simulink model "VOC"  (R2015a)
settings: Solver=ode3  StartTime=0.0  StopTime=3  FixedStep=Ts  RelTol=1e-3
values from neighbouring files (symbols this model uses):
  C = 2350e-6    (= 0.00235)    [VOC_param.m]    (also in VOC_param_paper.m = 0.0022; controller_parameters.m = 0.0022; power_control_param.m)
  Carrier_amp = 10    [VOC_param_paper.m]    (also in controller_parameters.m = 1)
  Ka = fluxeff    (= 0.15)    [VOC_param.m]    (also in VOC_param_paper.m; power_control_param.m)
  Kii = alphaI*R_hat    (= 628.318530718)    [VOC_param_paper.m]    (also in controller_parameters.m; current_controller_param.m = 1260)
  Kiv = 0.01    [VOC_param_paper.m]    (also in controller_parameters.m)
  Kpi = alphaI*L_hat    (= 37.6991118431)    [VOC_param_paper.m]    (also in controller_parameters.m; current_controller_param.m = 62.8)
  Kpv = alphaV*C_hat/(3*Vpcc_hat)    (= 0.0196071030862)    [VOC_param_paper.m]    (also in controller_parameters.m = alphaV*C_hat/(3*Vpcc_hat))
  L = 8e-3    (= 0.008)    [VOC_param.m]    (also in VOC_param_paper.m = 0.003; controller_parameters.m = 0.003; current_controller_param.m = 0.005; power_control_param.m)
  p = 4    [VOC_param.m]    (also in VOC_param_paper.m; power_control_param.m)
  R = 0.1    [VOC_param.m]    (also in VOC_param_paper.m = 0.05; controller_parameters.m = 0.05; current_controller_param.m; power_control_param.m)
  RL = 120    [VOC_param.m]    (also in VOC_param_paper.m = 150; power_control_param.m)
  rpm2radps = pi/30    (= 0.10471975512)    [VOC_param.m]    (also in VOC_param_paper.m; power_control_param.m)
  Ts = 1/fs    (= 1e-05)    [VOC_param.m]    (also in VOC_param_paper.m = 5e-05; controller_parameters.m = 5e-05; power_control_param.m)
  Udcref = 120    [VOC_param.m]    (also in VOC_param_paper.m; power_control_param.m = 100)
libraries: simulink x7, powerlib_meascontrol x6
settings Model: Creator=rblan  LastModifiedBy=rblan

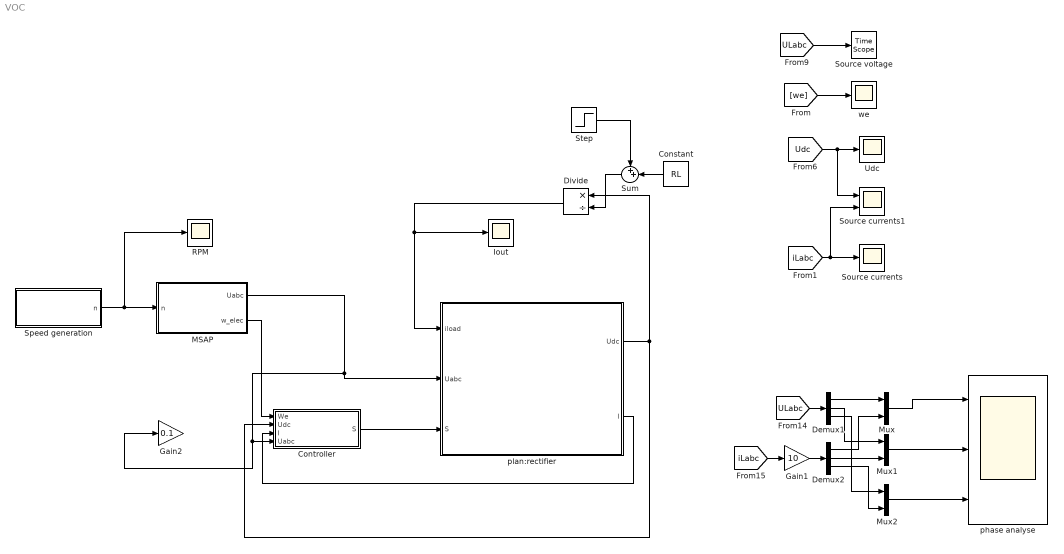
== system VOC ==
  Constant : Constant  Value=RL
  Controller : Subsystem
  Demux1 : Demux  Outputs=3
  Demux2 : Demux  Outputs=3
  Divide : Product  Inputs=*/
  Gain1 : Gain  Gain=10
  Gain2 : Gain  Gain=0.1
  Iout : Scope
      settings: YMin=0.2275  YMax=0.2575
  MSAP : Subsystem
  Mux : Mux  Inputs=2
  Mux1 : Mux  Inputs=2
  Mux2 : Mux  Inputs=2
  RPM : Scope
      settings: YMin=0.2275  YMax=0.2575  SaveName=ScopeData26
  Source currents : Scope
      settings: TimeRange=2  YMin=-11  YMax=11  SaveName=Iabc
  Source currents1 : Scope  NumInputPorts=2
      settings: TimeRange=2  YMin=-11~-5  YMax=11~5  SaveName=Iabc2
  "Source voltage " : TimeScope
  Speed generation : Subsystem
  Step : Step  Time=0.5  After=0  SampleTime=0
  Sum : Sum  Inputs=++|
  Udc : Scope
      settings: TimeRange=3  YMin=98.1  YMax=98.675  SaveName=Udc
  phase analyse : Scope  NumInputPorts=3
      settings: TimeRange=0.06239913932221623  YMin=-30~-30~-30  YMax=30~30~30  SaveName=Uabc2
  plan:rectifier : Subsystem
  we : Scope
      settings: YMin=119.381  YMax=131.947  SaveName=ScopeData10
  wires:
  [iLabc] -> Source currents1/2, Source currents/1
  [ULabc] -> "Source voltage "/1
  [we] -> we/1
  [ULabc] -> Demux1/1
  [iLabc] -> Gain1/1
  Mux/1 -> phase analyse/1
  Demux1/1 -> Mux/1
  Demux2/1 -> Mux/2
  Mux1/1 -> phase analyse/2
  Mux2/1 -> phase analyse/3
  Demux1/2 -> Mux1/1
  Demux2/2 -> Mux1/2
  Demux1/3 -> Mux2/1
  Demux2/3 -> Mux2/2
  Gain1/1 -> Demux2/1
  Speed generation/1(n) -> RPM/1, MSAP/1(n)
  MSAP/1(Uabc) -> Gain2/1, Controller/4(Uabc), plan:rectifier/2(Uabc)
  MSAP/2(w_elec) -> Controller/1(We)
  Controller/1(S) -> plan:rectifier/3(S)
  plan:rectifier/1(Udc) -> Controller/2(Udc), Divide/1
  Divide/1 -> plan:rectifier/1(iload), Iout/1
  Constant/1 -> Sum/2
  Step/1 -> Sum/1
  Sum/1 -> Divide/2
  plan:rectifier/2(I) -> Controller/3(I)
  [Udc] -> Source currents1/1, Udc/1

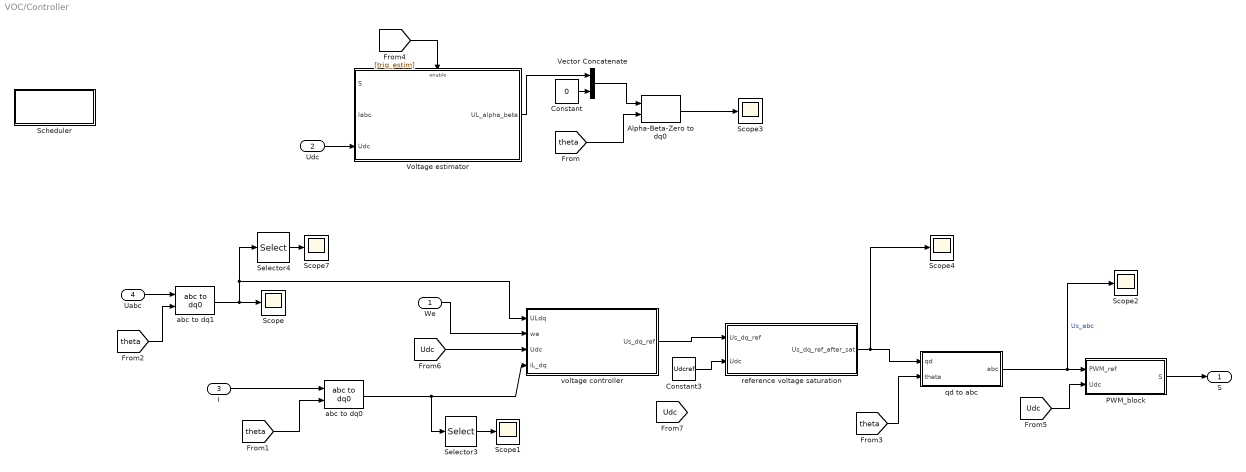
== system VOC/Controller ==
  We : Inport
  Udc : Inport  Port=2
  I : Inport  Port=3
  Uabc : Inport  Port=4
  Alpha-Beta-Zero to dq0 : powerlib_meascontrol/Transformations/Alpha-Beta-Zero to dq0  Alignment=Aligned with phase A axis
  Constant : Constant  Value=0
  Constant3 : Constant  Value=Udcref
  PWM_block : Subsystem
  Scheduler : Subsystem
  Scope{,1..4,7} (6 alike) : Scope
      Scope settings: YMin=-2.5  YMax=45
      Scope1 settings: YMin=-0.175  YMax=0.175  SaveName=ScopeData2
      Scope2 settings: YMin=-0.175  YMax=0.175  SaveName=ScopeData8
      Scope3 settings: YMin=-2.5  YMax=45  SaveName=ScopeData7
      Scope4 settings: YMin=-30  YMax=0  SaveName=ScopeData13
      Scope7 settings: YMin=-2.5  YMax=45  SaveName=ScopeData18
  Selector3 : Selector  InputPortWidth=3  Indices=[3]
  Selector4 : Selector  InputPortWidth=3  Indices=[3]
  Vector Concatenate : Concatenate
  Voltage estimator : Subsystem
  abc to dq0 : powerlib_meascontrol/Transformations/abc to dq0  Alignment=Aligned with phase A axis
  abc to dq1 : powerlib_meascontrol/Transformations/abc to dq0  Alignment=Aligned with phase A axis
  qd to abc : Subsystem
  reference voltage saturation : Subsystem
  voltage controller : Subsystem
  S : Outport
  wires:
  I/1 -> abc to dq0/1
  We/1 -> voltage controller/2(we)
  [theta] -> Alpha-Beta-Zero to dq0/2
  [theta] -> abc to dq0/2
  Voltage estimator/1(UL_alpha_beta) -> Vector Concatenate/1
  Vector Concatenate/1 -> Alpha-Beta-Zero to dq0/1
  Constant/1 -> Vector Concatenate/2
  Uabc/1 -> abc to dq1/1
  abc to dq1/1 -> voltage controller/1(ULdq), Selector4/1, Scope/1
  [theta] -> abc to dq1/2
  Alpha-Beta-Zero to dq0/1 -> Scope3/1
  [trig_estim] -> Voltage estimator/Enable
  abc to dq0/1 -> Selector3/1, voltage controller/4(iL_dq)
  Udc/1 -> Voltage estimator/3(Udc)
  Selector3/1 -> Scope1/1
  Selector4/1 -> Scope7/1
  [theta] -> qd to abc/2(theta)
  qd to abc/1(abc) -> Scope2/1, PWM_block/1(PWM_ref)  "Us_abc"
  PWM_block/1(S) -> S/1
  [Udc] -> PWM_block/2(Udc)
  [Udc] -> voltage controller/3(Udc)
  reference voltage saturation/1(Us_dq_ref_after_sat) -> Scope4/1, qd to abc/1(qd)
  voltage controller/1(Us_dq_ref) -> reference voltage saturation/1(Us_dq_ref)
  Constant3/1 -> reference voltage saturation/2("Udc ")

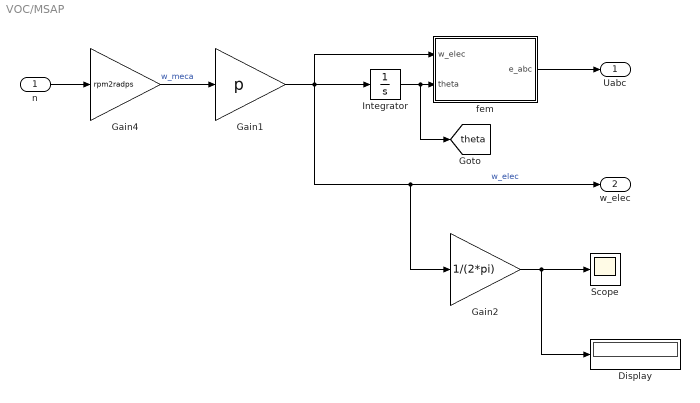
== system VOC/MSAP ==
  n : Inport
  Display : Display
  Gain1 : Gain  Gain=p
  Gain2 : Gain  Gain=1/(2*pi)
  Gain4 : Gain  Gain=rpm2radps
  Integrator : Integrator
  Scope : Scope
      settings: YMin=53.3333  YMax=53.3333  SaveName=ScopeData9
  fem : Subsystem
  Uabc : Outport
  w_elec : Outport  Port=2
  tag scope: theta=global
  wires:
  Integrator/1 -> [theta], fem/2(theta)
  Gain1/1 -> Integrator/1, Gain2/1, w_elec/1, fem/1(w_elec)  "w_elec"
  n/1 -> Gain4/1
  Gain4/1 -> Gain1/1  "w_meca"
  fem/1(e_abc) -> Uabc/1
  Gain2/1 -> Display/1, Scope/1

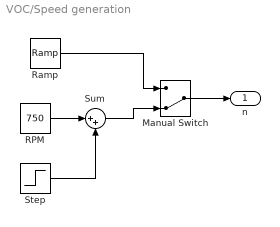
== system VOC/Speed generation ==
  Manual Switch : ManualSwitch  CurrentSetting=0
  RPM : Constant  Value=750
  Ramp : simulink/Sources/Ramp  slope=100  start=0  X0=700
  Step : Step  Time=0.5  After=0  SampleTime=0
  Sum : Sum  Inputs=|++
  n : Outport
  wires:
  Ramp/1 -> Manual Switch/1
  Manual Switch/1 -> n/1
  RPM/1 -> Sum/1
  Sum/1 -> Manual Switch/2
  Step/1 -> Sum/2

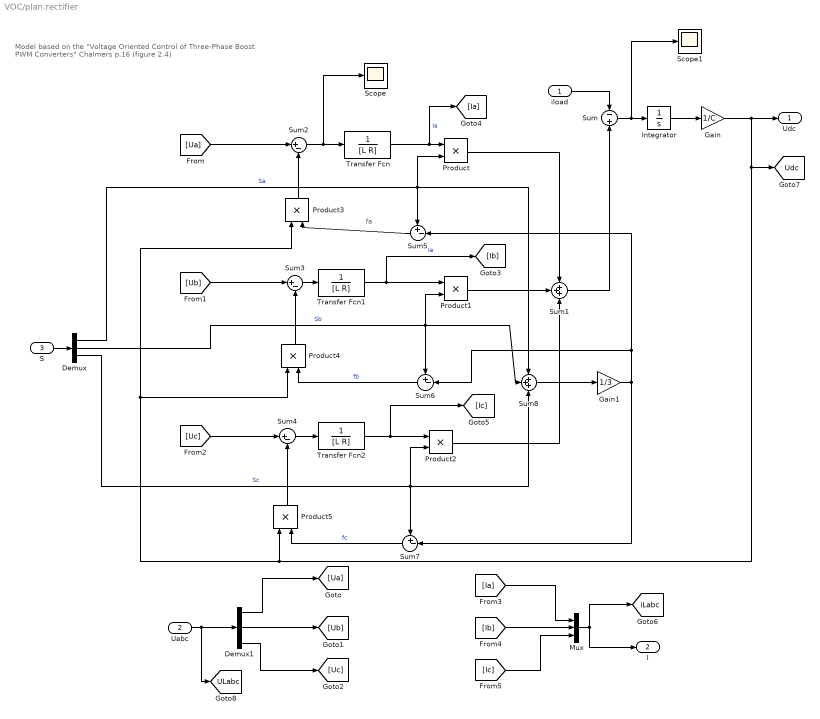
== system VOC/plan:rectifier ==
  note: fa
  note: Model based on the "Voltage Oriented Control of Three‐Phase
      | Boost PWM Converters" Chalmers p.16 (figure 2.4)
  iload : Inport
  Uabc : Inport  Port=2
  S : Inport  Port=3
  Demux : Demux  Outputs=3
  Demux1 : Demux  Outputs=3
  Gain : Gain  Gain=1/C
  Gain1 : Gain  Gain=1/3
  Integrator : Integrator
  Mux : Mux  Inputs=3
  Product{,1..5} (6 alike) : Product
  Scope : Scope
      settings: SaveName=ScopeData14
  Scope1 : Scope
      settings: SaveName=ScopeData12
  Sum : Sum  Inputs=-|+
  Sum1 : Sum  Inputs=+++
  Sum2 : Sum  Inputs=|+-
  Sum3 : Sum  Inputs=|+-
  Sum4 : Sum  Inputs=|+-
  Sum5 : Sum  Inputs=+-|
  Sum6 : Sum  Inputs=+-|
  Sum7 : Sum  Inputs=+-|
  Sum8 : Sum  Inputs=+++
  Transfer Fcn : TransferFcn  Denominator=[L R]  ContinuousStateAttributes='Ia'
  Transfer Fcn1 : TransferFcn  Denominator=[L R]
  Transfer Fcn2 : TransferFcn  Denominator=[L R]
  Udc : Outport
  I : Outport  Port=2
  tag scope: ULabc=global, Udc=global, iLabc=global
  wires:
  Gain/1 -> [Udc], Product5/1, Product3/1, Product4/1, Udc/1
  Integrator/1 -> Gain/1
  iload/1 -> Sum/1
  Sum1/1 -> Sum/2
  Product/1 -> Sum1/1
  Product1/1 -> Sum1/2
  Product2/1 -> Sum1/3
  Transfer Fcn/1 -> [Ia], Product/1  "Ia"
  Transfer Fcn1/1 -> [Ib], Product1/1  "Ia"
  Transfer Fcn2/1 -> [Ic], Product2/1
  Sum2/1 -> Scope/1, Transfer Fcn/1
  [Ua] -> Sum2/1
  Product3/1 -> Sum2/2
  Sum3/1 -> Transfer Fcn1/1
  Sum4/1 -> Transfer Fcn2/1
  [Ub] -> Sum3/1
  [Uc] -> Sum4/1
  Demux/1 -> Sum8/1, Product/2, Sum5/1  "Sa"
  Demux/2 -> Sum6/1, Sum8/2, Product1/2  "Sb"
  Demux/3 -> Sum8/3, Sum7/1, Product2/2  "Sc"
  Product4/1 -> Sum3/2
  Product5/1 -> Sum4/2
  Sum5/1 -> Product3/2
  Sum6/1 -> Product4/2  "fb"
  Sum7/1 -> Product5/2  "fc"
  Sum/1 -> Scope1/1, Integrator/1
  Sum8/1 -> Gain1/1
  Gain1/1 -> Sum6/2, Sum5/2, Sum7/2
  S/1 -> Demux/1
  Uabc/1 -> [ULabc], Demux1/1
  Demux1/1 -> [Ua]
  Demux1/2 -> [Ub]
  Demux1/3 -> [Uc]
  Mux/1 -> [iLabc], I/1
  [Ia] -> Mux/1
  [Ib] -> Mux/2
  [Ic] -> Mux/3

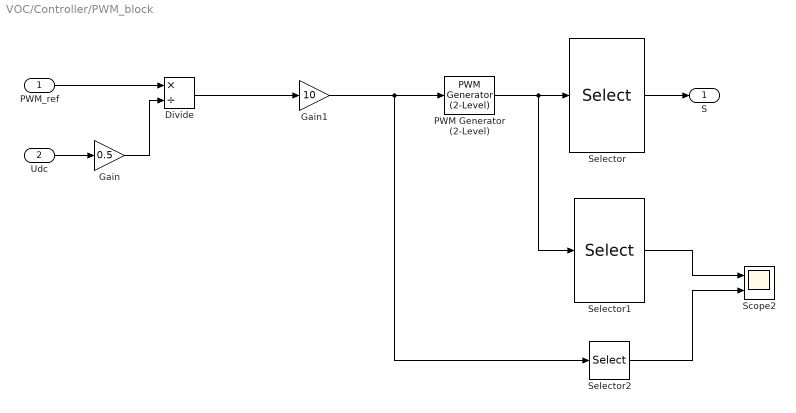
== system VOC/Controller/PWM_block ==
  PWM_ref : Inport
  Udc : Inport  Port=2
  Divide : Product  Inputs=*/
  Gain : Gain  Gain=0.5
  Gain1 : Gain  Gain=10
  PWM Generator (2-Level) : powerlib_meascontrol/Pulse & Signal Generators/PWM Generator (2-Level)  ModulatorType=Three-phase bridge (6 pulses)  ModulatorMode=Unsynchronized  Fc=Fsw  Pc=90  nF=27  MinMax="[-Carrier_amp  Carrier_amp]"  SamplingTechnique=Natural  ModulatingSignals=off  m=0.8  Freq=60  Phase=0  Ts=Ts  ShowCarrierOutport=off
  Scope2 : Scope  NumInputPorts=2
      settings: YMin=-22.499~-5  YMax=22.5254~5  SaveName=ScopeData3
  Selector : Selector  InputPortWidth=6  Indices=[1 3 5]
  Selector1 : Selector  InputPortWidth=6  Indices=[1]
  Selector2 : Selector  InputPortWidth=3  Indices=[1]
  S : Outport
  wires:
  PWM Generator (2-Level)/1 -> Selector1/1, Selector/1
  Gain/1 -> Divide/2
  Divide/1 -> Gain1/1
  Gain1/1 -> Selector2/1, PWM Generator (2-Level)/1
  PWM_ref/1 -> Divide/1
  Udc/1 -> Gain/1
  Selector/1 -> S/1
  Selector1/1 -> Scope2/1
  Selector2/1 -> Scope2/2

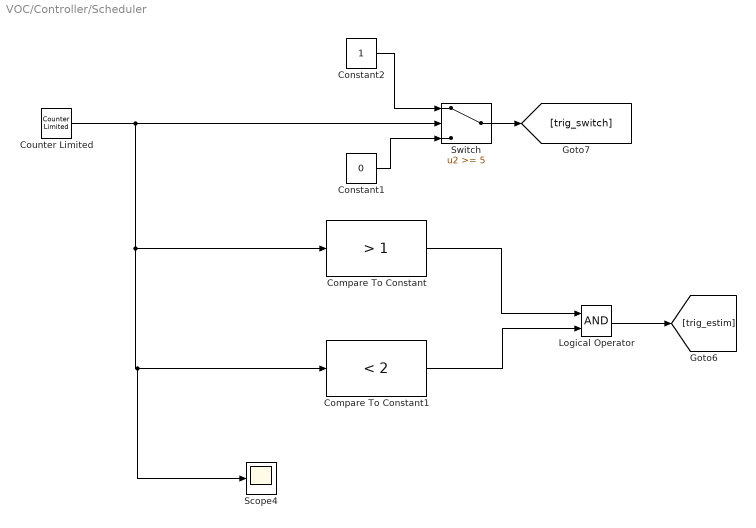
== system VOC/Controller/Scheduler ==
  Compare To Constant : simulink/Logic and Bit Operations/Compare To Constant  relop=>  const=1  OutDataTypeStr=boolean
  Compare To Constant1 : simulink/Logic and Bit Operations/Compare To Constant  relop=<  const=2  OutDataTypeStr=boolean
  Constant1 : Constant  Value=0
  Constant2 : Constant
  Counter Limited : simulink/Sources/Counter Limited  uplimit=5  tsamp=-1
  Logical Operator : Logic  AllPortsSameDT=off  OutDataTypeStr=boolean
  Scope4 : Scope
      settings: YMin=-275  YMax=175  SaveName=ScopeData23
  Switch : Switch  Threshold=5
  wires:
  Counter Limited/1 -> Compare To Constant/1, Scope4/1, Compare To Constant1/1, Switch/2
  Constant1/1 -> Switch/3
  Constant2/1 -> Switch/1
  Logical Operator/1 -> [trig_estim]
  Switch/1 -> [trig_switch]
  Compare To Constant/1 -> Logical Operator/1
  Compare To Constant1/1 -> Logical Operator/2

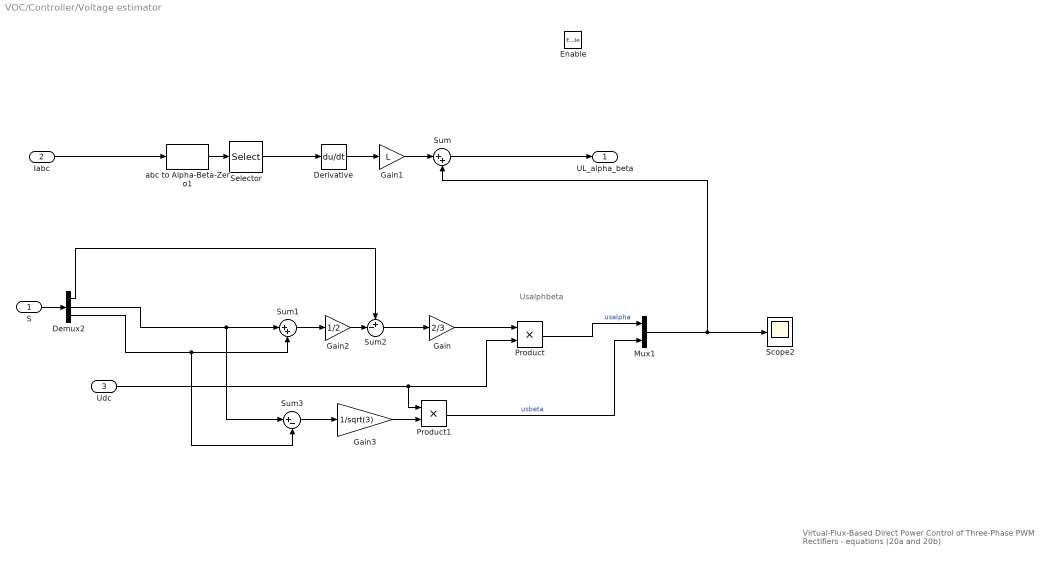
== system VOC/Controller/Voltage estimator ==
  note: Virtual-Flux-Based Direct Power Control of
      | Three-Phase PWM Rectifiers - equations (20a and 20b)
  note: Usalphbeta
  S : Inport
  Iabc : Inport  Port=2
  Udc : Inport  Port=3
  Enable : EnablePort
  Demux2 : Demux  Outputs=3
  Derivative : Derivative
  Gain : Gain  Gain=2/3
  Gain1 : Gain  Gain=L
  Gain2 : Gain  Gain=1/2
  Gain3 : Gain  Gain=1/sqrt(3)
  Mux1 : Mux  Inputs=2
  Product : Product
  Product1 : Product
  Scope2 : Scope
      settings: ShowLegends=on  YMin=-8  YMax=8  SaveName=ScopeData4
  Selector : Selector  InputPortWidth=3  Indices=[1 2]
  Sum : Sum  Inputs=|++
  Sum1 : Sum  Inputs=|++
  Sum2 : Sum  Inputs=+-|
  Sum3 : Sum  Inputs=|+-
  abc to Alpha-Beta-Zero1 : powerlib_meascontrol/Transformations/abc to Alpha-Beta-Zero
  UL_alpha_beta : Outport
  wires:
  abc to Alpha-Beta-Zero1/1 -> Selector/1
  Gain1/1 -> Sum/1
  Demux2/2 -> Sum3/1, Sum1/1
  Demux2/3 -> Sum3/2, Sum1/2
  Sum1/1 -> Gain2/1
  Gain2/1 -> Sum2/2
  Demux2/1 -> Sum2/1
  Sum2/1 -> Gain/1
  Gain/1 -> Product/1
  Udc/1 -> Product/2, Product1/1
  Product/1 -> Mux1/1  "usalpha"
  Sum3/1 -> Gain3/1
  Gain3/1 -> Product1/2
  Product1/1 -> Mux1/2  "usbeta"
  Mux1/1 -> Scope2/1, Sum/2
  S/1 -> Demux2/1
  Iabc/1 -> abc to Alpha-Beta-Zero1/1
  Derivative/1 -> Gain1/1
  Sum/1 -> UL_alpha_beta/1
  Selector/1 -> Derivative/1

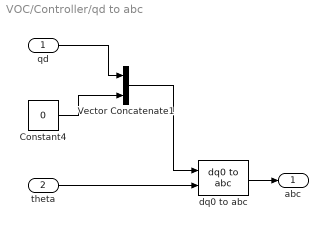
== system VOC/Controller/qd to abc ==
  qd : Inport
  theta : Inport  Port=2
  Constant4 : Constant  Value=0
  Vector Concatenate1 : Concatenate
  dq0 to abc : powerlib_meascontrol/Transformations/dq0 to abc  Alignment=Aligned with phase A axis
  abc : Outport
  wires:
  theta/1 -> dq0 to abc/2
  Vector Concatenate1/1 -> dq0 to abc/1
  qd/1 -> Vector Concatenate1/1
  Constant4/1 -> Vector Concatenate1/2
  dq0 to abc/1 -> abc/1

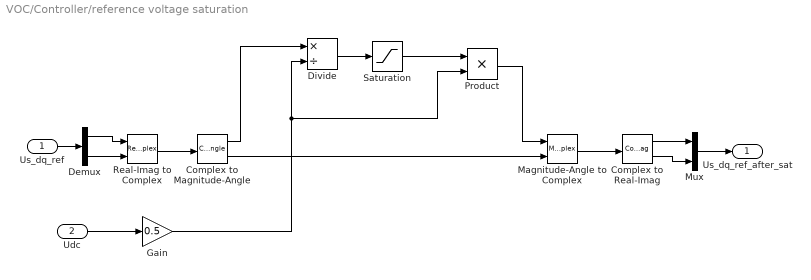
== system VOC/Controller/reference voltage saturation ==
  Us_dq_ref : Inport
  "Udc " : Inport  Port=2
  Complex to Magnitude-Angle : ComplexToMagnitudeAngle
  Complex to Real-Imag : ComplexToRealImag
  Demux : Demux  Outputs=2
  Divide : Product  Inputs=*/
  Gain : Gain  Gain=0.5
  Magnitude-Angle to Complex : MagnitudeAngleToComplex
  Mux : Mux  Inputs=2
  Product : Product
  Real-Imag to Complex : RealImagToComplex
  Saturation : Saturate
  Us_dq_ref_after_sat : Outport
  wires:
  Us_dq_ref/1 -> Demux/1
  Demux/1 -> Real-Imag to Complex/1
  Demux/2 -> Real-Imag to Complex/2
  "Udc "/1 -> Gain/1
  Mux/1 -> Us_dq_ref_after_sat/1
  Complex to Real-Imag/1 -> Mux/1
  Complex to Real-Imag/2 -> Mux/2
  Real-Imag to Complex/1 -> Complex to Magnitude-Angle/1
  Magnitude-Angle to Complex/1 -> Complex to Real-Imag/1
  Complex to Magnitude-Angle/2 -> Magnitude-Angle to Complex/2
  Divide/1 -> Saturation/1
  Saturation/1 -> Product/1
  Complex to Magnitude-Angle/1 -> Divide/1
  Gain/1 -> Product/2, Divide/2
  Product/1 -> Magnitude-Angle to Complex/1

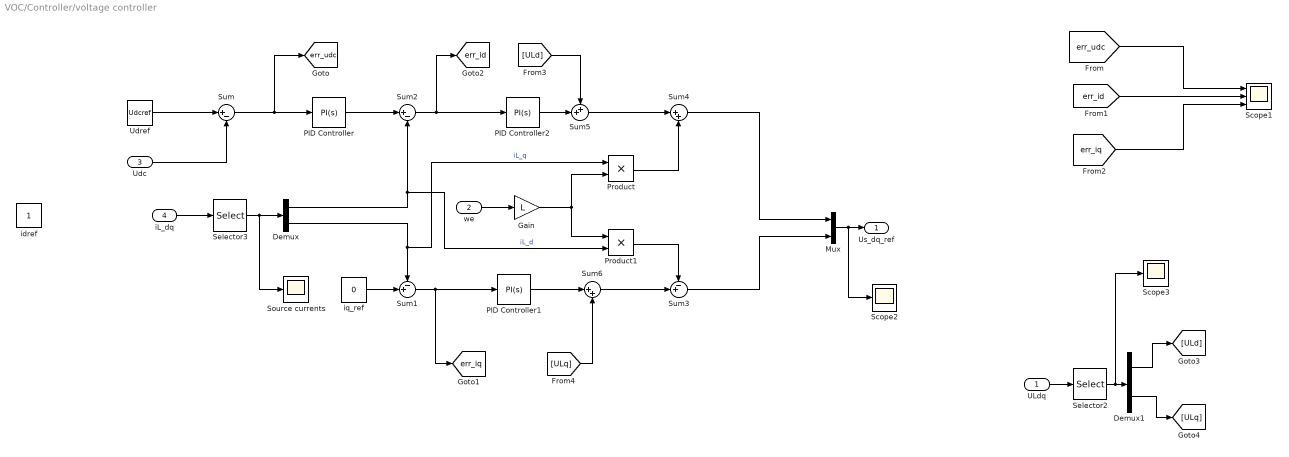
== system VOC/Controller/voltage controller ==
  ULdq : Inport
  we : Inport  Port=2
  Udc : Inport  Port=3
  iL_dq : Inport  Port=4
  Demux : Demux  Outputs=2
  Demux1 : Demux  Outputs=2
  Gain : Gain  Gain=L
  Mux : Mux  Inputs=2
  PID Controller : simulink/Continuous/PID Controller  Controller=PI  TimeDomain=Continuous-time  SampleTime=-1  IntegratorMethod=Forward Euler  FilterMethod=Forward Euler  Form=Parallel  UseFilter=on  ControllerParametersSource=internal  P=Kpv  I=Kiv  D=0  N=100  InitialConditionSource=internal  InitialConditionForIntegrator=0  InitialConditionForFilter=0  ExternalReset=none  LimitOutput=off  UpperSaturationLimit=inf  LowerSaturationLimit=-inf  LinearizeAsGain=on  AntiWindupMode=none  Kb=1  TrackingMode=off  Kt=1  PParamMin=[]  PParamMax=[]  IParamMin=[]  IParamMax=[]  DParamMin=[]  DParamMax=[]  NParamMin=[]  NParamMax=[]  KbParamMin=[]  KbParamMax=[]  KtParamMin=[]  KtParamMax=[]  POutMin=[]  POutMax=[]  IOutMin=[]  IOutMax=[]  DOutMin=[]  DOutMax=[]  NOutMin=[]  NOutMax=[]  KbOutMin=[]  KbOutMax=[]  KtOutMin=[]  KtOutMax=[]  IntegratorOutMin=[]  IntegratorOutMax=[]  FilterOutMin=[]  FilterOutMax=[]  SumOutMin=[]  SumOutMax=[]  SumI1OutMin=[]  SumI1OutMax=[]  SumI2OutMin=[]  SumI2OutMax=[]  SumI3OutMin=[]  SumI3OutMax=[]  SumDOutMin=[]  SumDOutMax=[]  SaturationOutMin=[]  SaturationOutMax=[]  IntegratorContinuousStateAttributes=''  IntegratorStateMustResolveToSignalObject=off  IntegratorRTWStateStorageClass=Auto  FilterContinuousStateAttributes=''  FilterStateMustResolveToSignalObject=off  FilterRTWStateStorageClass=Auto  DifferentiatorICPrevScaledInput=0  DifferentiatorOutMin=[]  DifferentiatorOutMax=[]
  PID Controller1 : simulink/Continuous/PID Controller  Controller=PI  TimeDomain=Continuous-time  SampleTime=-1  IntegratorMethod=Forward Euler  FilterMethod=Forward Euler  Form=Parallel  UseFilter=on  ControllerParametersSource=internal  P=Kpi  I=Kii  D=0  N=100  InitialConditionSource=internal  InitialConditionForIntegrator=0  InitialConditionForFilter=0  ExternalReset=none  LimitOutput=off  UpperSaturationLimit=inf  LowerSaturationLimit=-inf  LinearizeAsGain=on  AntiWindupMode=none  Kb=1  TrackingMode=off  Kt=1  PParamMin=[]  PParamMax=[]  IParamMin=[]  IParamMax=[]  DParamMin=[]  DParamMax=[]  NParamMin=[]  NParamMax=[]  KbParamMin=[]  KbParamMax=[]  KtParamMin=[]  KtParamMax=[]  POutMin=[]  POutMax=[]  IOutMin=[]  IOutMax=[]  DOutMin=[]  DOutMax=[]  NOutMin=[]  NOutMax=[]  KbOutMin=[]  KbOutMax=[]  KtOutMin=[]  KtOutMax=[]  IntegratorOutMin=[]  IntegratorOutMax=[]  FilterOutMin=[]  FilterOutMax=[]  SumOutMin=[]  SumOutMax=[]  SumI1OutMin=[]  SumI1OutMax=[]  SumI2OutMin=[]  SumI2OutMax=[]  SumI3OutMin=[]  SumI3OutMax=[]  SumDOutMin=[]  SumDOutMax=[]  SaturationOutMin=[]  SaturationOutMax=[]  IntegratorContinuousStateAttributes=''  IntegratorStateMustResolveToSignalObject=off  IntegratorRTWStateStorageClass=Auto  FilterContinuousStateAttributes=''  FilterStateMustResolveToSignalObject=off  FilterRTWStateStorageClass=Auto  DifferentiatorICPrevScaledInput=0  DifferentiatorOutMin=[]  DifferentiatorOutMax=[]
  PID Controller2 : simulink/Continuous/PID Controller  Controller=PI  TimeDomain=Continuous-time  SampleTime=-1  IntegratorMethod=Forward Euler  FilterMethod=Forward Euler  Form=Parallel  UseFilter=on  ControllerParametersSource=internal  P=Kpi  I=Kii  D=0  N=100  InitialConditionSource=internal  InitialConditionForIntegrator=0  InitialConditionForFilter=0  ExternalReset=none  LimitOutput=off  UpperSaturationLimit=inf  LowerSaturationLimit=-inf  LinearizeAsGain=on  AntiWindupMode=none  Kb=1  TrackingMode=off  Kt=1  PParamMin=[]  PParamMax=[]  IParamMin=[]  IParamMax=[]  DParamMin=[]  DParamMax=[]  NParamMin=[]  NParamMax=[]  KbParamMin=[]  KbParamMax=[]  KtParamMin=[]  KtParamMax=[]  POutMin=[]  POutMax=[]  IOutMin=[]  IOutMax=[]  DOutMin=[]  DOutMax=[]  NOutMin=[]  NOutMax=[]  KbOutMin=[]  KbOutMax=[]  KtOutMin=[]  KtOutMax=[]  IntegratorOutMin=[]  IntegratorOutMax=[]  FilterOutMin=[]  FilterOutMax=[]  SumOutMin=[]  SumOutMax=[]  SumI1OutMin=[]  SumI1OutMax=[]  SumI2OutMin=[]  SumI2OutMax=[]  SumI3OutMin=[]  SumI3OutMax=[]  SumDOutMin=[]  SumDOutMax=[]  SaturationOutMin=[]  SaturationOutMax=[]  IntegratorContinuousStateAttributes=''  IntegratorStateMustResolveToSignalObject=off  IntegratorRTWStateStorageClass=Auto  FilterContinuousStateAttributes=''  FilterStateMustResolveToSignalObject=off  FilterRTWStateStorageClass=Auto  DifferentiatorICPrevScaledInput=0  DifferentiatorOutMin=[]  DifferentiatorOutMax=[]
  Product : Product
  Product1 : Product
  Scope1 : Scope  NumInputPorts=3
      settings: YMin=-1~8.75~-2.4  YMax=3~12~-1.45  SaveName=ScopeData6
  Scope2 : Scope
      settings: TimeRange=1  YMin=-28  YMax=-6  SaveName=ScopeData11
  Scope3 : Scope
      settings: TimeRange=1  YMin=-28  YMax=-6  SaveName=ScopeData5
  Selector2 : Selector  InputPortWidth=3  Indices=[1 2]
  Selector3 : Selector  InputPortWidth=3  Indices=[1 2]
  Source currents : Scope
      settings: TimeRange=2  YMin=-2  YMax=11  SaveName=Iabc1
  Sum : Sum  Inputs=|+-
  Sum1 : Sum  Inputs=-+|
  Sum2 : Sum  Inputs=|+-
  Sum3 : Sum  Inputs=-+|
  Sum4 : Sum  Inputs=|++
  Sum5 : Sum  Inputs=++|
  Sum6 : Sum  Inputs=|++
  Udref : Constant  Value=Udcref
  idref : Constant
  iq_ref : Constant  Value=0
  Us_dq_ref : Outport
  tag scope: err_id=global, err_iq=global, err_udc=global
  wires:
  Sum1/1 -> [err_iq], PID Controller1/1
  Demux/2 -> Product/1, Sum1/1  "iL_q"
  Demux/1 -> Product1/2, Sum2/2  "iL_d"
  we/1 -> Gain/1
  iq_ref/1 -> Sum1/2
  Gain/1 -> Product1/1, Product/2
  Sum2/1 -> [err_id], PID Controller2/1
  Sum5/1 -> Sum4/1
  Sum4/1 -> Mux/1
  Sum3/1 -> Mux/2
  iL_dq/1 -> Selector3/1
  Mux/1 -> Scope2/1, Us_dq_ref/1
  Selector3/1 -> Source currents/1, Demux/1
  Udref/1 -> Sum/1
  Sum/1 -> [err_udc], PID Controller/1
  Udc/1 -> Sum/2
  PID Controller2/1 -> Sum5/2
  Product/1 -> Sum4/2
  Product1/1 -> Sum3/1
  Sum6/1 -> Sum3/2
  [err_udc] -> Scope1/1
  [err_id] -> Scope1/2
  [err_iq] -> Scope1/3
  ULdq/1 -> Selector2/1
  [ULd] -> Sum5/1
  Selector2/1 -> Scope3/1, Demux1/1
  Demux1/1 -> [ULd]
  Demux1/2 -> [ULq]
  PID Controller1/1 -> Sum6/1
  [ULq] -> Sum6/2
  PID Controller/1 -> Sum2/1

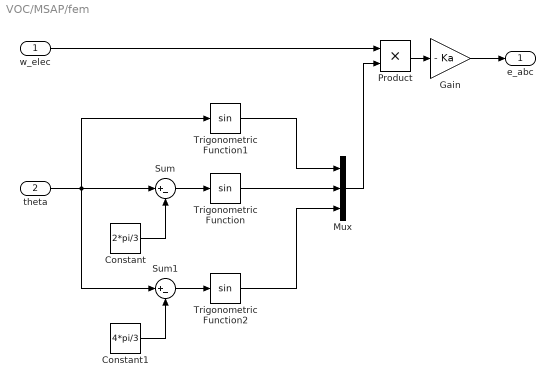
== system VOC/MSAP/fem ==
  w_elec : Inport
  theta : Inport  Port=2
  Constant : Constant  Value=2*pi/3
  Constant1 : Constant  Value=4*pi/3
  Gain : Gain  Gain=- Ka
  Mux : Mux  Inputs=3
  Product : Product
  Sum : Sum  Inputs=|+-
  Sum1 : Sum  Inputs=|+-
  Trigonometric Function : Trigonometry
  Trigonometric Function1 : Trigonometry
  Trigonometric Function2 : Trigonometry
  e_abc : Outport
  wires:
  Mux/1 -> Product/2
  theta/1 -> Sum/1, Trigonometric Function1/1, Sum1/1
  Constant1/1 -> Sum1/2
  Sum1/1 -> Trigonometric Function2/1
  Constant/1 -> Sum/2
  Sum/1 -> Trigonometric Function/1
  w_elec/1 -> Product/1
  Product/1 -> Gain/1
  Gain/1 -> e_abc/1
  Trigonometric Function1/1 -> Mux/1
  Trigonometric Function2/1 -> Mux/3
  Trigonometric Function/1 -> Mux/2
